simulink model "kinematicstest"  (R2018b)
settings: Solver=ode4  StartTime=0.0  StopTime=40  FixedStep=0.02  RelTol=1e-3
InitFcn:
  | kinematics_initial;
values from neighbouring files (symbols this model uses):
  b = 10.097    [kinematics_initial.m]
  cbar = 1.493520000000000    (= 1.49352)    [kinematics_initial.m]
  J = [948.0 0 0 ... (first row only)    [kinematics_initial.m]
  J_inv = inv(J)    [kinematics_initial.m]
  m = 1454.0*0.453592    (= 659.522768)    [kinematics_initial.m]
  omega_0 = [0;0;0]    [kinematics_initial.m]
  quaternion0 = angle2quat(euler0(3), euler0(2), euler0(1))    [kinematics_initial.m]
  VI0 = [40;0;0]    [kinematics_initial.m]
  XI0 = [0;0;-7]    [kinematics_initial.m]
undefined symbols (not defined in the file or in its folder): C172, current_CG_position, magnitude, QTG_C172
libraries: aerolibasang x3, aerolibtransform2 x2, aerolibatmos2 x2, sharedtransform x2, aerolibconvert2 x1, dspmtrx3 x1, sharedutil x1
settings Model: Creator=arthus  LastModifiedBy=arthus

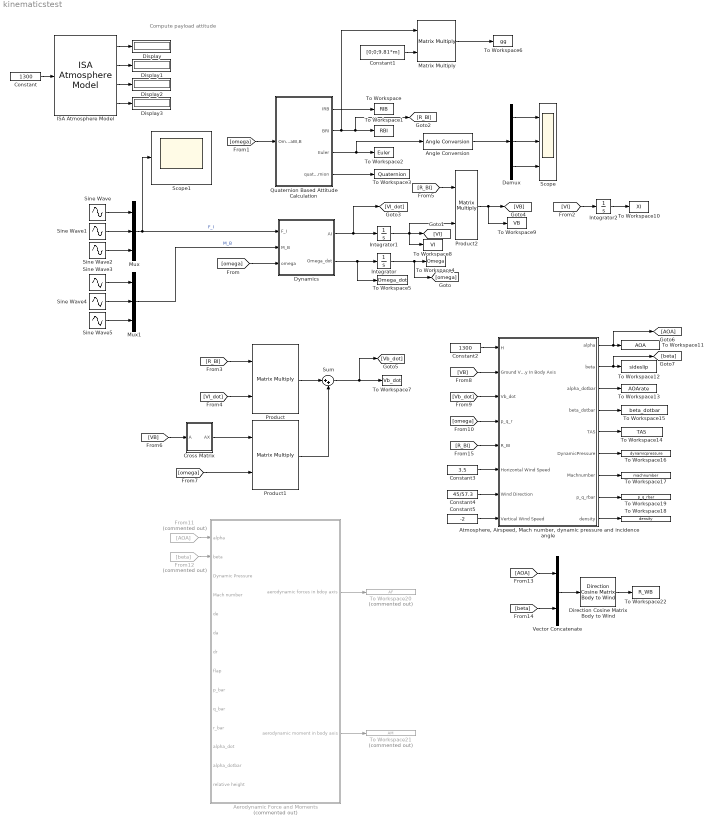
== system kinematicstest ==
  note: Compute payload attitude
  Aerodynamic Force and Moments : Subsystem  Commented=on
  Angle Conversion : aerolibconvert2/Angle Conversion  IU=rad  OU=deg
  "Atmosphere, Airspeed, Mach number, dynamic pressure and incidence angle " : Subsystem
  Constant : Constant  Value=1300
  Constant1 : Constant  Value=[0;0;9.81*m]  VectorParams1D=off
  Constant2 : Constant  Value=1300
  Constant3 : Constant  Value=3.5
  Constant4 : Constant  Value=45/57.3
  Constant5 : Constant  Value=-2
  Cross Matrix : Subsystem
  Demux : Demux  Outputs=3
  Direction Cosine Matrix Body to Wind : aerolibtransform2/Direction Cosine Matrix Body to Wind
      settings: SourceProductName=Aerospace Blockset  SourceProductBaseCode=AE
  Display{,1..3} (4 alike) : Display
  Dynamics : Subsystem
  From11 : From  Commented=on  GotoTag=AOA
  From12 : From  Commented=on  GotoTag=beta
  ISA Atmosphere Model : aerolibatmos2/ISA Atmosphere Model  custom=off  g=9.80665  gamma=1.4  R=287.0531  L=0.0065  h_trop=11000  h_strat=20000  rho0=1.225  P0=101325  T0=288.15  h0=0
      settings: SourceProductName=Aerospace Blockset
  Integrator : Integrator  InitialCondition=omega_0
  Integrator1 : Integrator  InitialCondition=VI0
  Integrator2 : Integrator  InitialCondition=XI0
  Matrix Multiply : Product  Multiplication=Matrix(*)
  Mux : Mux  Inputs=3
  Mux1 : Mux  Inputs=3
  Product : Product  Multiplication=Matrix(*)
  Product1 : Product  Multiplication=Matrix(*)
  Product2 : Product  Multiplication=Matrix(*)
  Quaternion Based Attitude Calculation : Subsystem
  Scope : Scope  NumInputPorts=3
  Scope1 : Scope
  Sine Wave : Sin  Amplitude=0.3  Frequency=pi  SampleTime=0
  Sine Wave1 : Sin  Amplitude=0.1  Frequency=pi  SampleTime=0
  Sine Wave2 : Sin  Amplitude=0.4  Frequency=pi  SampleTime=0
  Sine Wave3 : Sin  Amplitude=0.3  Frequency=pi  SampleTime=0
  Sine Wave4 : Sin  Amplitude=0.1  Frequency=pi  SampleTime=0
  Sine Wave5 : Sin  Amplitude=0.4  Frequency=pi  SampleTime=0
  Sum : Sum  Inputs=|++
  To Workspace : ToWorkspace  VariableName=RIB  SampleTime=-1
  To Workspace1 : ToWorkspace  VariableName=RBI  SampleTime=-1
  To Workspace10 : ToWorkspace  VariableName=XI  SampleTime=-1
  To Workspace11 : ToWorkspace  VariableName=AOA  SampleTime=-1
  To Workspace12 : ToWorkspace  VariableName=sideslip  SampleTime=-1
  To Workspace13 : ToWorkspace  VariableName=AOArate  SampleTime=-1
  To Workspace14 : ToWorkspace  VariableName=TAS  SampleTime=-1
  To Workspace15 : ToWorkspace  VariableName=beta_dotbar  SampleTime=-1
  To Workspace16 : ToWorkspace  VariableName=dynamicpressure  SampleTime=-1
  To Workspace17 : ToWorkspace  VariableName=machnumber  SampleTime=-1
  To Workspace18 : ToWorkspace  VariableName=density  SampleTime=-1
  To Workspace19 : ToWorkspace  VariableName=p_q_rbar  SampleTime=-1
  To Workspace2 : ToWorkspace  VariableName=Euler  SampleTime=-1
  To Workspace20 : ToWorkspace  Commented=on  VariableName=AF  SampleTime=-1
  To Workspace21 : ToWorkspace  Commented=on  VariableName=AM  SampleTime=-1
  To Workspace22 : ToWorkspace  VariableName=R_WB  SampleTime=-1
  To Workspace3 : ToWorkspace  VariableName=Quaternion  SampleTime=-1
  To Workspace4 : ToWorkspace  VariableName=Omega  SampleTime=-1
  To Workspace5 : ToWorkspace  VariableName=Omega_dot  SampleTime=-1
  To Workspace6 : ToWorkspace  VariableName=gg  SampleTime=-1
  To Workspace7 : ToWorkspace  VariableName=Vb_dot  SampleTime=-1
  To Workspace8 : ToWorkspace  VariableName=VI  SampleTime=-1
  To Workspace9 : ToWorkspace  VariableName=VB  SampleTime=-1
  Vector Concatenate : Concatenate
  wires:
  Quaternion Based Attitude Calculation/3(Euler) -> Angle Conversion/1, To Workspace2/1
  Quaternion Based Attitude Calculation/2(BRI) -> Matrix Multiply/1, [R_BI], To Workspace1/1
  Quaternion Based Attitude Calculation/1(IRB) -> To Workspace/1
  Quaternion Based Attitude Calculation/4(quaternion) -> To Workspace3/1
  Sine Wave/1 -> Mux/1
  Sine Wave1/1 -> Mux/2
  Sine Wave2/1 -> Mux/3
  Demux/1 -> Scope/1
  Demux/2 -> Scope/2
  Demux/3 -> Scope/3
  Angle Conversion/1 -> Demux/1
  Constant/1 -> ISA Atmosphere Model/1
  ISA Atmosphere Model/1 -> Display/1
  ISA Atmosphere Model/2 -> Display1/1
  ISA Atmosphere Model/3 -> Display2/1
  ISA Atmosphere Model/4 -> Display3/1
  Constant1/1 -> Matrix Multiply/2
  Matrix Multiply/1 -> To Workspace6/1
  Dynamics/1(AI) -> [VI_dot], Integrator1/1
  Dynamics/2(Omega_dot) -> To Workspace5/1, Integrator/1
  Integrator1/1 -> To Workspace8/1, Product2/2, [VI]
  Integrator/1 -> [omega], To Workspace4/1
  Mux/1 -> Scope1/1, Dynamics/1(F_I)  "F_I"
  [omega] -> Dynamics/3(omega)
  Sine Wave5/1 -> Mux1/3
  Sine Wave3/1 -> Mux1/1
  Sine Wave4/1 -> Mux1/2
  Mux1/1 -> Dynamics/2(M_B)  "M_B"
  [omega] -> Quaternion Based Attitude Calculation/1(OmegaBI,B)
  [VI_dot] -> Product/2
  [R_BI] -> Product/1
  Product/1 -> Sum/1
  Sum/1 -> [Vb_dot], To Workspace7/1
  Cross Matrix/1(AX) -> Product1/1
  [R_BI] -> Product2/1
  Product2/1 -> To Workspace9/1, [VB]
  [VB] -> Cross Matrix/1(A)
  [omega] -> Product1/2
  Product1/1 -> Sum/2
  [VI] -> Integrator2/1
  Integrator2/1 -> To Workspace10/1
  Constant2/1 -> "Atmosphere, Airspeed, Mach number, dynamic pressure and incidence angle "/1(H)
  [VB] -> "Atmosphere, Airspeed, Mach number, dynamic pressure and incidence angle "/2(Ground Velocity In Body Axis)
  [Vb_dot] -> "Atmosphere, Airspeed, Mach number, dynamic pressure and incidence angle "/3(Vb_dot)
  [omega] -> "Atmosphere, Airspeed, Mach number, dynamic pressure and incidence angle "/4(p_q_r)
  "Atmosphere, Airspeed, Mach number, dynamic pressure and incidence angle "/1(alpha) -> [AOA], To Workspace11/1
  "Atmosphere, Airspeed, Mach number, dynamic pressure and incidence angle "/2(beta) -> [beta], To Workspace12/1
  "Atmosphere, Airspeed, Mach number, dynamic pressure and incidence angle "/3(alpha_dotbar) -> To Workspace13/1
  "Atmosphere, Airspeed, Mach number, dynamic pressure and incidence angle "/5(TAS) -> To Workspace14/1
  "Atmosphere, Airspeed, Mach number, dynamic pressure and incidence angle "/4(beta_dotbar) -> To Workspace15/1
  "Atmosphere, Airspeed, Mach number, dynamic pressure and incidence angle "/6(DynamicPressure) -> To Workspace16/1
  "Atmosphere, Airspeed, Mach number, dynamic pressure and incidence angle "/7(Machnumber) -> To Workspace17/1
  "Atmosphere, Airspeed, Mach number, dynamic pressure and incidence angle "/9(density) -> To Workspace18/1
  "Atmosphere, Airspeed, Mach number, dynamic pressure and incidence angle "/8(p_q_rbar) -> To Workspace19/1
  Aerodynamic Force and Moments/1(aerodynamic forces in bdoy axis) -> To Workspace20/1
  Aerodynamic Force and Moments/2(aerodynamic moment in body axis) -> To Workspace21/1
  From11/1 -> Aerodynamic Force and Moments/1(alpha)
  From12/1 -> Aerodynamic Force and Moments/2(beta)
  Vector Concatenate/1 -> Direction Cosine Matrix Body to Wind/1
  [AOA] -> Vector Concatenate/1
  [beta] -> Vector Concatenate/2
  Direction Cosine Matrix Body to Wind/1 -> To Workspace22/1
  [R_BI] -> "Atmosphere, Airspeed, Mach number, dynamic pressure and incidence angle "/5(R_BI)
  Constant3/1 -> "Atmosphere, Airspeed, Mach number, dynamic pressure and incidence angle "/6(Horizontal Wind Speed)
  Constant4/1 -> "Atmosphere, Airspeed, Mach number, dynamic pressure and incidence angle "/7(Wind Direction)
  Constant5/1 -> "Atmosphere, Airspeed, Mach number, dynamic pressure and incidence angle "/8(Vertical Wind Speed)

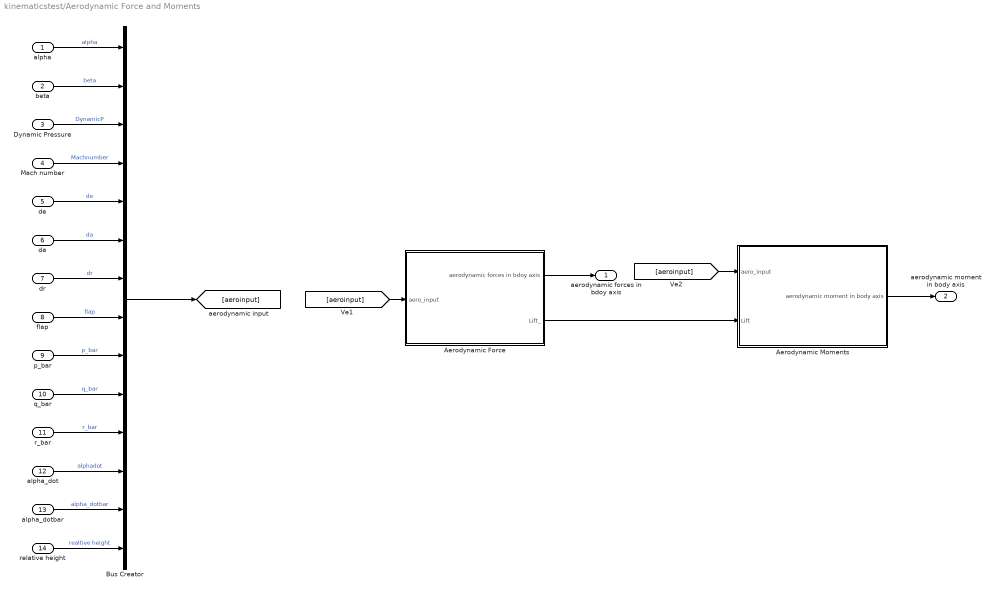
== system kinematicstest/Aerodynamic Force and Moments ==
  alpha : Inport
  beta : Inport  Port=2
  Dynamic Pressure : Inport  Port=3
  Mach number : Inport  Port=4
  de : Inport  Port=5
  da : Inport  Port=6
  dr : Inport  Port=7
  flap : Inport  Port=8
  p_bar : Inport  Port=9
  q_bar : Inport  Port=10
  r_bar : Inport  Port=11
  alpha_dot : Inport  Port=12
  alpha_dotbar : Inport  Port=13
  relative height : Inport  Port=14
  "Aerodynamic Force " : Subsystem  mask(Calculate Aerodynamic Forces in body axis){referenceaera=C172.Geometry.wingarea}
      mask prompts: referenceaera "Wing Aera"
  Aerodynamic Moments : Subsystem  mask(Calculate Aerodynamic Moments in body axis){referenceaera=C172.Geometry.wingarea, meanchord=C172.Geometry.chord, span=C172.Geometry.wingspan}
  Bus Creator : BusCreator  Inputs=14
  aerodynamic forces in bdoy axis : Outport
  aerodynamic moment in body axis : Outport  Port=2
  wires:
  alpha/1 -> Bus Creator/1  "alpha"
  beta/1 -> Bus Creator/2  "beta"
  Dynamic Pressure/1 -> Bus Creator/3  "DynamicP"
  Mach number/1 -> Bus Creator/4  "Machnumber"
  de/1 -> Bus Creator/5  "de"
  da/1 -> Bus Creator/6  "da"
  dr/1 -> Bus Creator/7  "dr"
  flap/1 -> Bus Creator/8  "flap"
  Bus Creator/1 -> [aeroinput]
  p_bar/1 -> Bus Creator/9  "p_bar"
  q_bar/1 -> Bus Creator/10  "q_bar"
  r_bar/1 -> Bus Creator/11  "r_bar"
  alpha_dot/1 -> Bus Creator/12  "alphadot"
  alpha_dotbar/1 -> Bus Creator/13  "alpha_dotbar"
  "Aerodynamic Force "/1(aerodynamic forces in bdoy axis) -> aerodynamic forces in bdoy axis/1
  Aerodynamic Moments/1(aerodynamic moment in body axis) -> aerodynamic moment in body axis/1
  [aeroinput] -> "Aerodynamic Force "/1(aero_input)
  [aeroinput] -> Aerodynamic Moments/1(aero_input)
  relative height/1 -> Bus Creator/14  "realtive height"
  "Aerodynamic Force "/2(Lift_) -> Aerodynamic Moments/2(Lift)

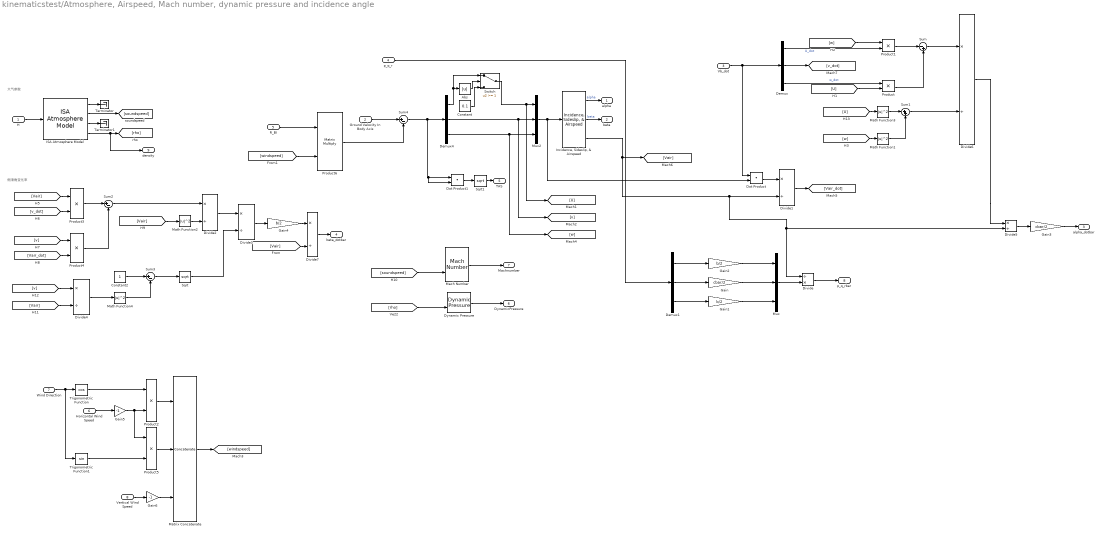
== system kinematicstest/Atmosphere, Airspeed, Mach number, dynamic pressure and incidence angle  ==
  note: 侧滑角变化率
  note: 大气参数
  H : Inport
  Ground Velocity In Body Axis : Inport  Port=2
  Vb_dot : Inport  Port=3
  p_q_r : Inport  Port=4
  R_BI : Inport  Port=5
  Horizontal Wind Speed : Inport  Port=6
  Wind Direction : Inport  Port=7
  Vertical Wind Speed : Inport  Port=8
  Abs : Abs
  Constant : Constant  Value=0.1
  Constant2 : Constant
  Demux : Demux  Outputs=3
  Demux1 : Demux  Outputs=3
  Demux4 : Demux  Outputs=3
  Divide : Product  Inputs=/*
  Divide{1..7} (7 alike) : Product  Inputs=*/
  Dot Product : DotProduct  InputSameDT=on  OutDataTypeStr=Inherit: Inherit via internal rule
  Dot Product1 : DotProduct  InputSameDT=on  OutDataTypeStr=Inherit: Inherit via internal rule
  Dynamic Pressure : aerolibasang/Dynamic Pressure
  Gain : Gain  Gain=cbar/2
  Gain1 : Gain  Gain=b/2
  Gain2 : Gain  Gain=b/2
  Gain3 : Gain  Gain=cbar/2
  Gain4 : Gain  Gain=b/2
  Gain5 : Gain  Gain=-1
  Gain6 : Gain  Gain=-1
  ISA Atmosphere Model : aerolibatmos2/ISA Atmosphere Model  custom=off  g=9.80665  gamma=1.4  R=287.0531  L=0.0065  h_trop=11000  h_strat=20000  rho0=1.225  P0=101325  T0=288.15  h0=0
      settings: SourceProductName=Aerospace Blockset
  "Incidence, Sideslip, & Airspeed" : aerolibasang/Incidence, Sideslip, & Airspeed
      settings: SourceProductName=Aerospace Blockset
  Mach Number : aerolibasang/Mach Number
      settings: SourceProductName=Aerospace Blockset  SourceProductBaseCode=AE
  Math Function{1..4} (4 alike) : Math  Operator=magnitude^2  SaturateOnIntegerOverflow=on
  Matrix Concatenate : Concatenate  NumInputs=3  Mode=Multidimensional array
  Mux : Mux  Inputs=3
  Mux2 : Mux  Inputs=3
  Product{,1,3..4} (4 alike) : Product  RndMeth=Zero
  Product2 : Product
  Product5 : Product
  Product6 : Product  Multiplication=Matrix(*)
  Sqrt : Sqrt  SaturateOnIntegerOverflow=on
  Sqrt1 : Sqrt  SaturateOnIntegerOverflow=on
  Sum : Sum  Inputs=|-+
  Sum1 : Sum  Inputs=|++
  Sum2 : Sum  Inputs=|+-
  Sum3 : Sum  Inputs=|+-
  Sum4 : Sum  Inputs=|+-
  Switch : Switch  Threshold=1
  Terminator : Terminator
  Terminator1 : Terminator
  Trigonometric Function : Trigonometry  Operator=cos
  Trigonometric Function1 : Trigonometry
  alpha : Outport
  beta : Outport  Port=2
  alpha_dotbar : Outport  Port=3
  beta_dotbar : Outport  Port=4
  TAS : Outport  Port=5
  DynamicPressure : Outport  Port=6
  Machnumber : Outport  Port=7
  p_q_rbar : Outport  Port=8
  density : Outport  Port=9
  wires:
  "Incidence, Sideslip, & Airspeed"/2 -> beta/1  "beta"
  "Incidence, Sideslip, & Airspeed"/1 -> alpha/1  "alpha"
  "Incidence, Sideslip, & Airspeed"/3 -> Divide1/2, Divide/1, Divide5/2, [Vair]
  Mux2/1 -> "Incidence, Sideslip, & Airspeed"/1, Dot Product/2
  Demux4/2 -> Mux2/2, [v]
  Demux4/3 -> Mux2/3, [w]
  Abs/1 -> Switch/2
  Switch/1 -> Mux2/1, [U]
  Demux4/1 -> Abs/1, Switch/1
  Constant/1 -> Switch/3
  ISA Atmosphere Model/1 -> Terminator/1
  ISA Atmosphere Model/3 -> Terminator1/1
  ISA Atmosphere Model/2 -> [soundspeed]
  ISA Atmosphere Model/4 -> density/1, [rho]
  H/1 -> ISA Atmosphere Model/1
  [soundspeed] -> Mach Number/2
  Mach Number/1 -> Machnumber/1
  Dynamic Pressure/1 -> DynamicPressure/1
  [rho] -> Dynamic Pressure/2
  Demux/1 -> Product1/2  "U_dot"
  Demux/2 -> [v_dot]
  Demux/3 -> Product/1  "w_dot"
  [U] -> Product/2
  Product/1 -> Sum/2
  [w] -> Product1/1
  Product1/1 -> Sum/1
  Sum/1 -> Divide6/1
  Math Function3/1 -> Sum1/1
  [Vair] -> Product3/1
  [v_dot] -> Product3/2
  Product3/1 -> Sum2/1
  [v] -> Product4/1
  [Vair_dot] -> Product4/2
  Product4/1 -> Sum2/2
  Dot Product/1 -> Divide1/1
  Divide1/1 -> [Vair_dot]
  Sum2/1 -> Divide2/1
  Math Function2/1 -> Divide2/2
  [Vair] -> Math Function2/1
  Divide2/1 -> Divide3/1
  Sqrt/1 -> Divide3/2
  Sum3/1 -> Sqrt/1
  Constant2/1 -> Sum3/1
  Math Function4/1 -> Sum3/2
  Divide4/1 -> Math Function4/1
  [Vair] -> Divide4/2
  [v] -> Divide4/1
  Divide3/1 -> Gain4/1
  [U] -> Math Function3/1
  Sum1/1 -> Divide6/2
  [w] -> Math Function1/1
  Math Function1/1 -> Sum1/2
  Vb_dot/1 -> Demux/1, Dot Product/1
  Dot Product1/1 -> Sqrt1/1
  Sqrt1/1 -> TAS/1
  Demux1/2 -> Gain/1
  Demux1/3 -> Gain1/1
  Demux1/1 -> Gain2/1
  Gain2/1 -> Mux/1
  Gain/1 -> Mux/2
  Gain1/1 -> Mux/3
  Mux/1 -> Divide/2
  Divide/1 -> p_q_rbar/1
  Divide5/1 -> Gain3/1
  Gain3/1 -> alpha_dotbar/1
  p_q_r/1 -> Demux1/1
  Divide6/1 -> Divide5/1
  Gain4/1 -> Divide7/1
  Divide7/1 -> beta_dotbar/1
  [Vair] -> Divide7/2
  R_BI/1 -> Product6/1
  Wind Direction/1 -> Trigonometric Function1/1, Trigonometric Function/1
  Trigonometric Function/1 -> Product2/1
  Horizontal Wind Speed/1 -> Gain5/1
  Trigonometric Function1/1 -> Product5/2
  Gain5/1 -> Product5/1, Product2/2
  Vertical Wind Speed/1 -> Gain6/1
  Product2/1 -> Matrix Concatenate/1
  Product5/1 -> Matrix Concatenate/2
  Gain6/1 -> Matrix Concatenate/3
  Matrix Concatenate/1 -> [windspeed]
  [windspeed] -> Product6/2
  Sum4/1 -> Dot Product1/2, Dot Product1/1, Demux4/1
  Product6/1 -> Sum4/2
  Ground Velocity In Body Axis/1 -> Sum4/1

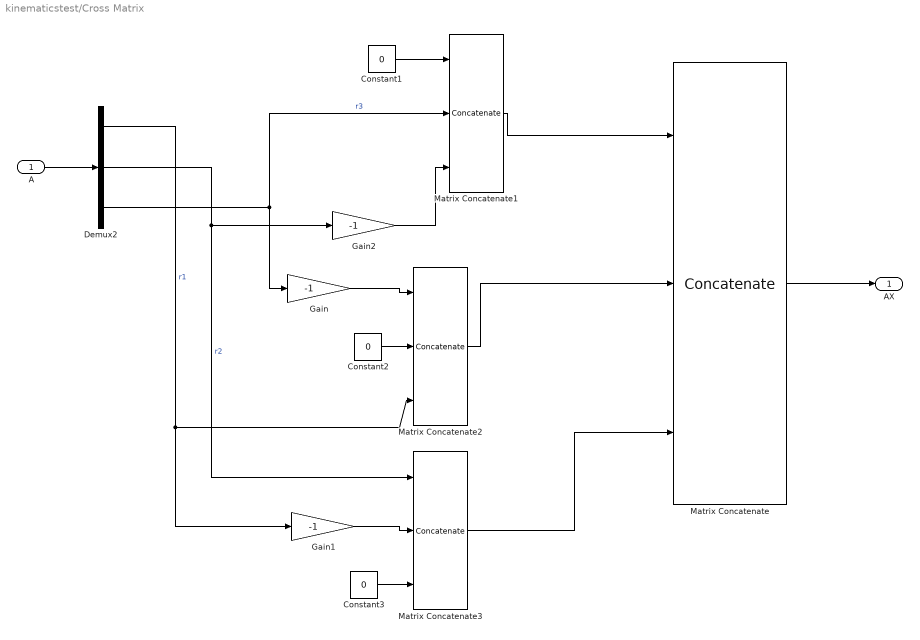
== system kinematicstest/Cross Matrix ==
  A : Inport
  Constant1 : Constant  Value=0  VectorParams1D=off
  Constant2 : Constant  Value=0  VectorParams1D=off
  Constant3 : Constant  Value=0  VectorParams1D=off
  Demux2 : Demux  Outputs=3
  Gain : Gain  Gain=-1
  Gain1 : Gain  Gain=-1
  Gain2 : Gain  Gain=-1
  Matrix Concatenate : Concatenate  NumInputs=3  Mode=Multidimensional array  ConcatenateDimension=2
  Matrix Concatenate1 : Concatenate  NumInputs=3  Mode=Multidimensional array
  Matrix Concatenate2 : Concatenate  NumInputs=3  Mode=Multidimensional array
  Matrix Concatenate3 : Concatenate  NumInputs=3  Mode=Multidimensional array
  AX : Outport
  wires:
  A/1 -> Demux2/1
  Demux2/1 -> Gain1/1, Matrix Concatenate2/3  "r1"
  Demux2/2 -> Gain2/1, Matrix Concatenate3/1  "r2"
  Matrix Concatenate/1 -> AX/1
  Demux2/3 -> Gain/1, Matrix Concatenate1/2  "r3"
  Matrix Concatenate1/1 -> Matrix Concatenate/1
  Matrix Concatenate2/1 -> Matrix Concatenate/2
  Constant2/1 -> Matrix Concatenate2/2
  Gain/1 -> Matrix Concatenate2/1
  Matrix Concatenate3/1 -> Matrix Concatenate/3
  Gain1/1 -> Matrix Concatenate3/2
  Constant3/1 -> Matrix Concatenate3/3
  Constant1/1 -> Matrix Concatenate1/1
  Gain2/1 -> Matrix Concatenate1/3

== system kinematicstest/Dynamics ==
  F_I : Inport
  M_B : Inport  Port=2
  omega : Inport  Port=3
  Cross Matrix : Subsystem
  Gain : Gain  Gain=1/m
  Gain1 : Gain  Gain=J_inv  Multiplication=Matrix(K*u)
  Gain2 : Gain  Gain=J  Multiplication=Matrix(K*u)
  Product : Product  Multiplication=Matrix(*)
  Sum : Sum  Inputs=|+-
  AI : Outport
  Omega_dot : Outport  Port=2
  wires:
  Gain/1 -> AI/1
  F_I/1 -> Gain/1
  Sum/1 -> Gain1/1
  Gain1/1 -> Omega_dot/1
  M_B/1 -> Sum/1
  omega/1 -> Product/2, Cross Matrix/1(A)
  Cross Matrix/1(AX) -> Gain2/1
  Gain2/1 -> Product/1
  Product/1 -> Sum/2

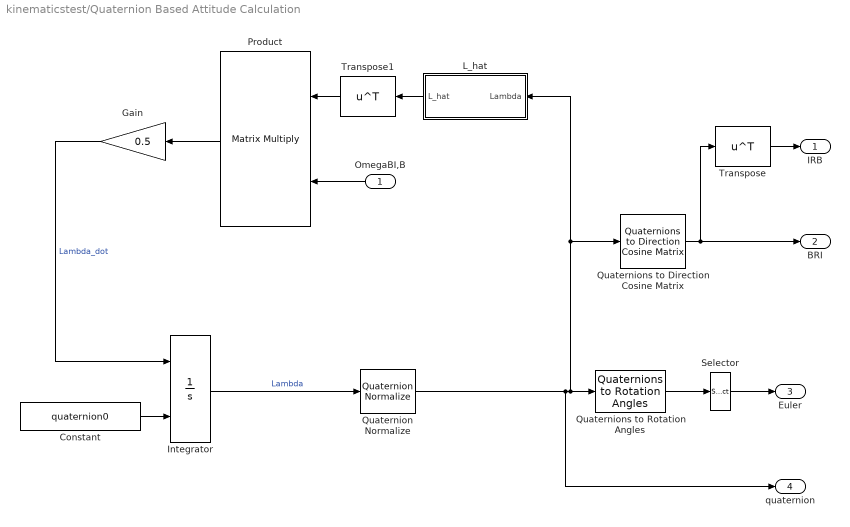
== system kinematicstest/Quaternion Based Attitude Calculation ==
  OmegaBI,B : Inport
  Constant : Constant  Value=quaternion0
  Gain : Gain  Gain=0.5
  Integrator : Integrator  InitialConditionSource=external
  L_hat : Subsystem
  Product : Product  Multiplication=Matrix(*)  RndMeth=Zero
  Quaternion Normalize : sharedutil/Quaternion Normalize  aMode=aMode
      settings: SourceProductName=Aerospace Blockset  SourceProductBaseCode=AE
  Quaternions to Direction Cosine Matrix : sharedtransform/Quaternions to  Direction Cosine Matrix  aMode=aMode
      settings: SourceProductName=Aerospace Blockset  SourceProductBaseCode=AE
  Quaternions to Rotation Angles : sharedtransform/Quaternions to Rotation Angles  rotationOrder=ZYX  aMode=aMode
      settings: SourceProductBaseCode=AE
  Selector : Selector  InputPortWidth=3  IndexOptions=Index vector (dialog)  Indices=[3 2 1]  OutputSizes=1
  Transpose : Math  Operator=transpose  SaturateOnIntegerOverflow=on
  Transpose1 : Math  Operator=transpose  SaturateOnIntegerOverflow=on
  IRB : Outport
  BRI : Outport  Port=2
  Euler : Outport  Port=3
  quaternion : Outport  Port=4
  wires:
  Constant/1 -> Integrator/2
  Quaternions to Rotation Angles/1 -> Selector/1
  Selector/1 -> Euler/1
  Integrator/1 -> Quaternion Normalize/1  "Lambda"
  Gain/1 -> Integrator/1  "Lambda_dot"
  Quaternions to Direction Cosine Matrix/1 -> BRI/1, Transpose/1
  Transpose/1 -> IRB/1
  L_hat/1(L_hat) -> Transpose1/1
  Transpose1/1 -> Product/1
  OmegaBI,B/1 -> Product/2
  Product/1 -> Gain/1
  Quaternion Normalize/1 -> Quaternions to Rotation Angles/1, Quaternions to Direction Cosine Matrix/1, L_hat/1(Lambda), quaternion/1

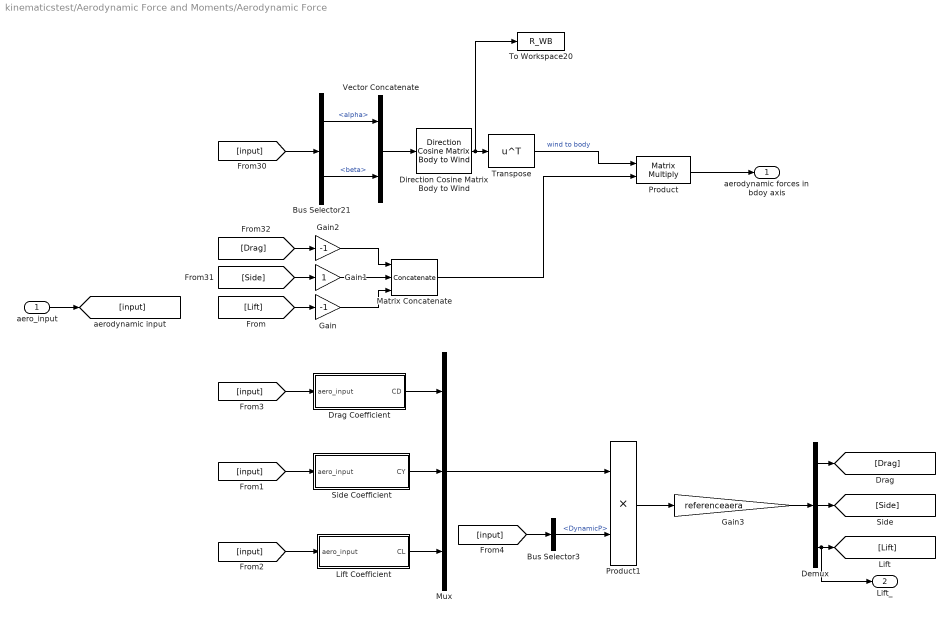
== system kinematicstest/Aerodynamic Force and Moments/Aerodynamic Force  ==
  aero_input : Inport
  Bus Selector21 : BusSelector  OutputSignals=alpha,beta
  Bus Selector3 : BusSelector  OutputSignals=DynamicP
  Demux : Demux  Outputs=3
  Direction Cosine Matrix Body to Wind : aerolibtransform2/Direction Cosine Matrix Body to Wind
      settings: SourceProductName=Aerospace Blockset  SourceProductBaseCode=AE
  Drag Coefficient : Subsystem
  Gain : Gain  Gain=-1
  Gain1 : Gain
  Gain2 : Gain  Gain=-1
  Gain3 : Gain  Gain=referenceaera
  Lift Coefficient : Subsystem
  Matrix Concatenate : Concatenate  NumInputs=3  Mode=Multidimensional array
  Mux : Mux  Inputs=3
  Product : Product  Multiplication=Matrix(*)  RndMeth=Zero
  Product1 : Product  RndMeth=Zero
  Side Coefficient : Subsystem
  To Workspace20 : ToWorkspace  VariableName=R_WB  SampleTime=-1
  Transpose : Math  Operator=transpose  SaturateOnIntegerOverflow=on
  Vector Concatenate : Concatenate
  aerodynamic forces in bdoy axis : Outport
  Lift_ : Outport  Port=2
  wires:
  Transpose/1 -> Product/1  "wind to body"
  Direction Cosine Matrix Body to Wind/1 -> To Workspace20/1, Transpose/1
  Matrix Concatenate/1 -> Product/2
  Gain2/1 -> Matrix Concatenate/1
  [Drag] -> Gain2/1
  Gain1/1 -> Matrix Concatenate/2
  [Side] -> Gain1/1
  Gain/1 -> Matrix Concatenate/3
  [Lift] -> Gain/1
  Vector Concatenate/1 -> Direction Cosine Matrix Body to Wind/1
  Bus Selector21/1 -> Vector Concatenate/1  "<alpha>"
  Bus Selector21/2 -> Vector Concatenate/2  "<beta>"
  [input] -> Bus Selector21/1
  aero_input/1 -> [input]
  [input] -> Bus Selector3/1
  Bus Selector3/1 -> Product1/2  "<DynamicP>"
  Product1/1 -> Gain3/1
  Mux/1 -> Product1/1
  Gain3/1 -> Demux/1
  Demux/1 -> [Drag]
  Demux/2 -> [Side]
  Demux/3 -> Lift_/1, [Lift]
  Product/1 -> aerodynamic forces in bdoy axis/1
  Drag Coefficient/1(CD) -> Mux/1
  Side Coefficient/1(CY) -> Mux/2
  [input] -> Lift Coefficient/1(aero_input)
  [input] -> Side Coefficient/1(aero_input)
  Lift Coefficient/1(CL) -> Mux/3
  [input] -> Drag Coefficient/1(aero_input)

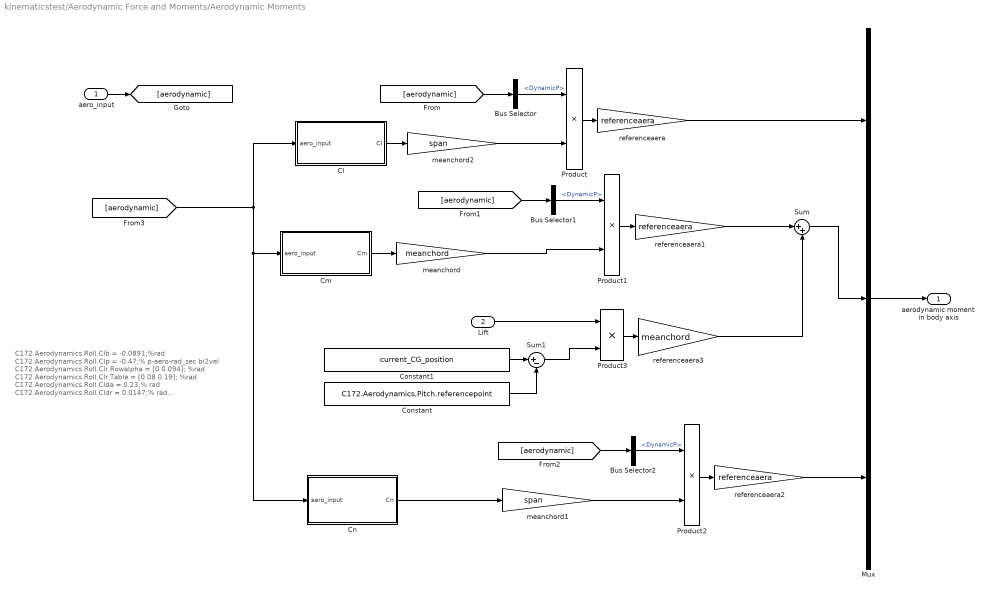
== system kinematicstest/Aerodynamic Force and Moments/Aerodynamic Moments ==
  note: C172.Aerodynamics.Roll.Clb = -0.0891;%rad
      | C172.Aerodynamics.Roll.Clp = -0.47;% p-aero-rad_sec bi2vel
      | C172.Aerodynamics.Roll.Clr.Rowalpha = [0 0.094];  %rad
      | C172.Aerodynamics.Roll.Clr.Table = [0.08 0.19];   %rad
      | C172.Aerodynamics.Roll.Clda = 0.23;% rad
      | C172.Aerodynamics.Roll.Cldr = 0.0147;% rad
      | C172.Aerodynamics.Pitch.Cmalpha = -1.8;% alpha-rad
      | C172.Aerodynamics.Pitch.CmDf.RowFlap = [0 10 20 30];%deg
      | C172.Aerodynamics.Pitch.CmDf.Table = [0 -0.03 -0.05 -0.06];%
      | C172.Aerodynamics.Pitch.CmDf.Type = 'Delta Pitch Moment';
      | C172.Aerodynamics.Pitch.Cmq = -12.4; % q-aero-rad_sec ci2vel
      | C172.Aerodynamics.Pitch.Cmadot = -5.2; % alphadot-rad_sec
      | C172.Aerodynamics.Pitch.Cm0 = 0.1; %
      | C172.Aerodynamics.Pitch.Cmde = -1.28; % elevator-pos-rad
      | C172.Aerodynamics.Yaw.Cnb = 0.0650;% rad
      | C172.Aerodynamics.Yaw.Cnp = -0.03;% p-aero-rad_sec bi2vel
      | C172.Aerodynamics.Yaw.Cnr = -0.099;%  r-aero-rad_sec bi2vel
      | C172.Aerodynamics.Yaw.Cnda = 0.0053;% rad
      | C172.Aerodynamics.Yaw.Cndr = -0.043;% rad
  aero_input : Inport
  Lift : Inport  Port=2
  Bus Selector : BusSelector  OutputSignals=DynamicP
  Bus Selector1 : BusSelector  OutputSignals=DynamicP
  Bus Selector2 : BusSelector  OutputSignals=DynamicP
  Cl : Subsystem
  Cm : Subsystem
  Cn : Subsystem
  Constant : Constant  Value=C172.Aerodynamics.Pitch.referencepoint
  Constant1 : Constant  Value=current_CG_position
  Mux : Mux  Inputs=3
  Product : Product  RndMeth=Zero
  Product1 : Product  RndMeth=Zero
  Product2 : Product  RndMeth=Zero
  Product3 : Product
  Sum : Sum  Inputs=|++
  Sum1 : Sum  Inputs=|+-
  meanchord : Gain  Gain=meanchord
  meanchord1 : Gain  Gain=span
  meanchord2 : Gain  Gain=span
  referenceaera : Gain  Gain=referenceaera
  referenceaera1 : Gain  Gain=referenceaera
  referenceaera2 : Gain  Gain=referenceaera
  referenceaera3 : Gain  Gain=meanchord
  aerodynamic moment in body axis : Outport
  wires:
  Product/1 -> referenceaera/1
  Bus Selector/1 -> Product/1  "<DynamicP>"
  Cn/1(Cn) -> meanchord1/1
  aero_input/1 -> [aerodynamic]
  Cm/1(Cm) -> meanchord/1
  [aerodynamic] -> Cn/1(aero_input), Cm/1(aero_input), Cl/1(aero_input)
  Cl/1(Cl) -> meanchord2/1
  [aerodynamic] -> Bus Selector/1
  Mux/1 -> aerodynamic moment in body axis/1
  meanchord2/1 -> Product/2
  referenceaera/1 -> Mux/1
  Product1/1 -> referenceaera1/1
  Bus Selector1/1 -> Product1/1  "<DynamicP>"
  [aerodynamic] -> Bus Selector1/1
  meanchord/1 -> Product1/2
  Product2/1 -> referenceaera2/1
  Bus Selector2/1 -> Product2/1  "<DynamicP>"
  [aerodynamic] -> Bus Selector2/1
  referenceaera1/1 -> Sum/1
  Sum/1 -> Mux/2
  referenceaera3/1 -> Sum/2
  referenceaera2/1 -> Mux/3
  meanchord1/1 -> Product2/2
  Constant1/1 -> Sum1/1
  Constant/1 -> Sum1/2
  Product3/1 -> referenceaera3/1
  Lift/1 -> Product3/1
  Sum1/1 -> Product3/2

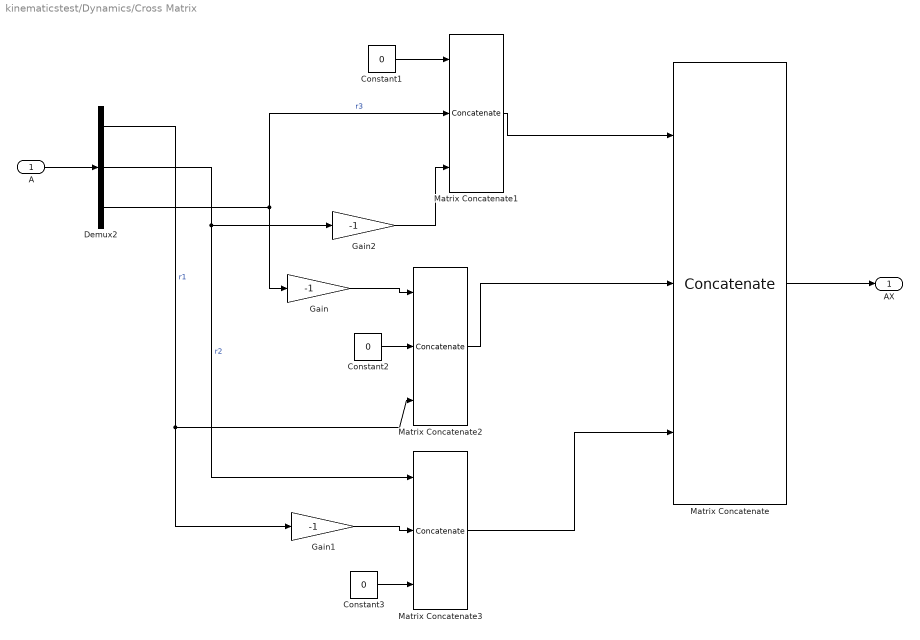
== system kinematicstest/Dynamics/Cross Matrix ==
  A : Inport
  Constant1 : Constant  Value=0  VectorParams1D=off
  Constant2 : Constant  Value=0  VectorParams1D=off
  Constant3 : Constant  Value=0  VectorParams1D=off
  Demux2 : Demux  Outputs=3
  Gain : Gain  Gain=-1
  Gain1 : Gain  Gain=-1
  Gain2 : Gain  Gain=-1
  Matrix Concatenate : Concatenate  NumInputs=3  Mode=Multidimensional array  ConcatenateDimension=2
  Matrix Concatenate1 : Concatenate  NumInputs=3  Mode=Multidimensional array
  Matrix Concatenate2 : Concatenate  NumInputs=3  Mode=Multidimensional array
  Matrix Concatenate3 : Concatenate  NumInputs=3  Mode=Multidimensional array
  AX : Outport
  wires:
  A/1 -> Demux2/1
  Demux2/1 -> Gain1/1, Matrix Concatenate2/3  "r1"
  Demux2/2 -> Gain2/1, Matrix Concatenate3/1  "r2"
  Matrix Concatenate/1 -> AX/1
  Demux2/3 -> Gain/1, Matrix Concatenate1/2  "r3"
  Matrix Concatenate1/1 -> Matrix Concatenate/1
  Matrix Concatenate2/1 -> Matrix Concatenate/2
  Constant2/1 -> Matrix Concatenate2/2
  Gain/1 -> Matrix Concatenate2/1
  Matrix Concatenate3/1 -> Matrix Concatenate/3
  Gain1/1 -> Matrix Concatenate3/2
  Constant3/1 -> Matrix Concatenate3/3
  Constant1/1 -> Matrix Concatenate1/1
  Gain2/1 -> Matrix Concatenate1/3

== system kinematicstest/Quaternion Based Attitude Calculation/L_hat ==
  Lambda : Inport
  Create Diagonal Matrix : dspmtrx3/Create Diagonal Matrix
      settings: SourceProductName=DSP System Toolbox  SourceProductBaseCode=DS
  Cross Matrix : Subsystem
  Gain : Gain  Gain=-1
  Gain1 : Gain  Gain=[1 1 1]
  Gain2 : Gain  Gain=-1
  Matrix Concatenate : Concatenate  Mode=Multidimensional array  ConcatenateDimension=2
  Selector : Selector  InputPortWidth=4  IndexOptions=Index vector (dialog)  Indices=[2 3 4]  OutputSizes=1
  Selector1 : Selector  InputPortWidth=4  IndexOptions=Index vector (dialog)  Indices=[1]  OutputSizes=1
  Sum : Sum  Inputs=|++
  L_hat : Outport
  wires:
  Lambda/1 -> Selector/1, Selector1/1
  Gain/1 -> Matrix Concatenate/1
  Matrix Concatenate/1 -> L_hat/1
  Cross Matrix/1(AX) -> Gain2/1  "LambdaX"
  Sum/1 -> Matrix Concatenate/2
  Selector1/1 -> Gain1/1
  Gain1/1 -> Create Diagonal Matrix/1
  Selector/1 -> Cross Matrix/1(A), Gain/1
  Create Diagonal Matrix/1 -> Sum/2
  Gain2/1 -> Sum/1

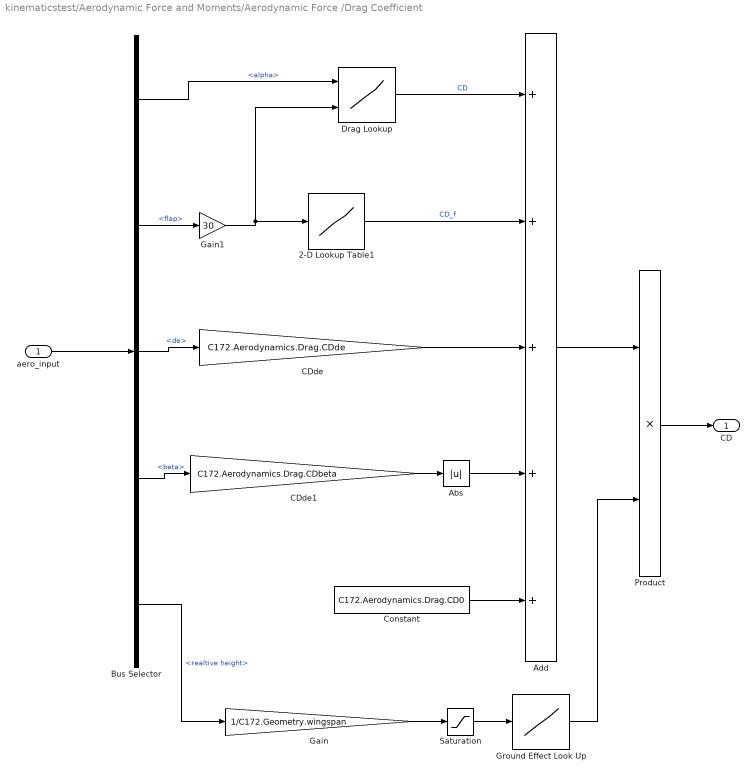
== system kinematicstest/Aerodynamic Force and Moments/Aerodynamic Force /Drag Coefficient ==
  aero_input : Inport
  2-D Lookup Table1 : Lookup_n-D  NumberOfTableDimensions=1  BreakpointsForDimension1=C172.Aerodynamics.Drag.CDDf.RowFlap  BreakpointsForDimension2=C172.Aerodynamics.Drag.CDwbh.ColumnFlap  Table=C172.Aerodynamics.Drag.CDDf.Table  InternalRulePriority=Speed  RndMeth=Simplest  InputSameDT=on
  Abs : Abs
  Add : Sum  Inputs=+++++
  Bus Selector : BusSelector  OutputSignals=alpha,flap,de,beta,realtive height
  CDde : Gain  Gain=C172.Aerodynamics.Drag.CDde
  CDde1 : Gain  Gain=C172.Aerodynamics.Drag.CDbeta
  Constant : Constant  Value=C172.Aerodynamics.Drag.CD0
  Drag Lookup : Lookup_n-D  BreakpointsForDimension1=C172.Aerodynamics.Drag.CDwbh.RowAlpha  BreakpointsForDimension2=C172.Aerodynamics.Drag.CDwbh.ColumnFlap  Table=C172.Aerodynamics.Drag.CDwbh.Table  InternalRulePriority=Speed  RndMeth=Simplest  InputSameDT=on
  Gain : Gain  Gain=1/C172.Geometry.wingspan
  Gain1 : Gain  Gain=30
  Ground Effect Look Up : Lookup_n-D  NumberOfTableDimensions=1  BreakpointsForDimension1=C172.Aerodynamics.GroundDragEffect.RowHeight  BreakpointsForDimension2=C172.Aerodynamics.Drag.CDwbh.ColumnFlap  Table=C172.Aerodynamics.GroundDragEffect.Table  InternalRulePriority=Speed  RndMeth=Simplest  InputSameDT=on
  Product : Product
  Saturation : Saturate  UpperLimit=1.1  LowerLimit=0
  CD : Outport
  wires:
  Drag Lookup/1 -> Add/1  "CD"
  aero_input/1 -> Bus Selector/1
  Constant/1 -> Add/5
  2-D Lookup Table1/1 -> Add/2  "CD_f"
  CDde1/1 -> Abs/1
  CDde/1 -> Add/3
  Bus Selector/3 -> CDde/1  "<de>"
  Bus Selector/4 -> CDde1/1  "<beta>"
  Abs/1 -> Add/4
  Bus Selector/2 -> Gain1/1  "<flap>"
  Bus Selector/1 -> Drag Lookup/1  "<alpha>"
  Add/1 -> Product/1
  Product/1 -> CD/1
  Ground Effect Look Up/1 -> Product/2
  Bus Selector/5 -> Gain/1  "<realtive height>"
  Saturation/1 -> Ground Effect Look Up/1
  Gain/1 -> Saturation/1
  Gain1/1 -> Drag Lookup/2, 2-D Lookup Table1/1

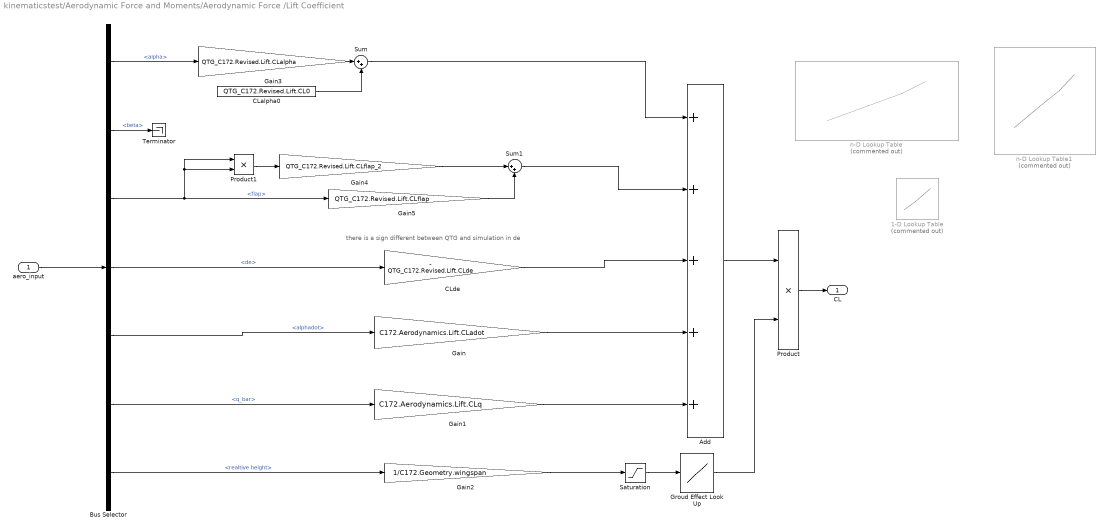
== system kinematicstest/Aerodynamic Force and Moments/Aerodynamic Force /Lift Coefficient ==
  note: there is a sign different between QTG and simulation in de
  aero_input : Inport
  1-D Lookup Table : Lookup_n-D  Commented=on  NumberOfTableDimensions=1  BreakpointsForDimension1=C172.Aerodynamics.Lift.CLDf.RowFlap  Table=C172.Aerodynamics.Lift.CLDf.Table  InternalRulePriority=Speed  RndMeth=Simplest  InputSameDT=on
  Add : Sum  Inputs=+++++
  Bus Selector : BusSelector  OutputSignals=alpha,beta,flap,de,alphadot,q_bar,realtive height
  CLalpha0 : Constant  Value=QTG_C172.Revised.Lift.CL0
  CLde : Gain  Gain=- QTG_C172.Revised.Lift.CLde
  Gain : Gain  Gain=C172.Aerodynamics.Lift.CLadot
  Gain1 : Gain  Gain=C172.Aerodynamics.Lift.CLq
  Gain2 : Gain  Gain=1/C172.Geometry.wingspan
  Gain3 : Gain  Gain=QTG_C172.Revised.Lift.CLalpha
  Gain4 : Gain  Gain=QTG_C172.Revised.Lift.CLflap_2
  Gain5 : Gain  Gain=QTG_C172.Revised.Lift.CLflap
  Groud Effect Look Up : Lookup_n-D  NumberOfTableDimensions=1  BreakpointsForDimension1=C172.Aerodynamics.GroundLiftEffect.RowHeight  Table=C172.Aerodynamics.GroundLiftEffect.Table  InternalRulePriority=Speed  RndMeth=Simplest  InputSameDT=on
  Product : Product
  Product1 : Product
  Saturation : Saturate  UpperLimit=1.1  LowerLimit=0
  Sum : Sum  Inputs=|++
  Sum1 : Sum  Inputs=|++
  Terminator : Terminator
  n-D Lookup Table : Lookup_n-D  Commented=on  BreakpointsForDimension1=C172.Aerodynamics.Lift.CLwbh.RowAlpha  BreakpointsForDimension2=C172.Aerodynamics.Lift.CLwbh.Stall_Hyst_Norm  BreakpointsForDimension3=[5, 7]  Table=C172.Aerodynamics.Lift.CLwbh.Table  InternalRulePriority=Speed  RndMeth=Simplest  InputSameDT=on
  n-D Lookup Table1 : Lookup_n-D  Commented=on  NumberOfTableDimensions=3  BreakpointsForDimension1=C172.Aerodynamics.Lift.CLalpha.RowAlpha  BreakpointsForDimension2=C172.Aerodynamics.Lift.CLalpha.ColumnBeta  BreakpointsForDimension3=C172.Aerodynamics.Lift.CLalpha.PageFlap  Table=C172.Aerodynamics.Lift.CLalpha.Table  InternalRulePriority=Speed  RndMeth=Simplest  InputSameDT=on
  CL : Outport
  wires:
  aero_input/1 -> Bus Selector/1
  Bus Selector/6 -> Gain1/1  "<q_bar>"
  Gain1/1 -> Add/5
  Bus Selector/5 -> Gain/1  "<alphadot>"
  Gain/1 -> Add/4
  Bus Selector/4 -> CLde/1  "<de>"
  CLde/1 -> Add/3
  Add/1 -> Product/1
  Product/1 -> CL/1
  Groud Effect Look Up/1 -> Product/2
  Gain2/1 -> Saturation/1
  Saturation/1 -> Groud Effect Look Up/1
  Bus Selector/7 -> Gain2/1  "<realtive height>"
  Sum/1 -> Add/1
  CLalpha0/1 -> Sum/2
  Bus Selector/1 -> Gain3/1  "<alpha>"
  Gain3/1 -> Sum/1
  Bus Selector/2 -> Terminator/1  "<beta>"
  Bus Selector/3 -> Product1/2, Product1/1, Gain5/1  "<flap>"
  Sum1/1 -> Add/2
  Gain4/1 -> Sum1/1
  Gain5/1 -> Sum1/2
  Product1/1 -> Gain4/1

== system kinematicstest/Aerodynamic Force and Moments/Aerodynamic Force /Side Coefficient ==
  aero_input : Inport
  Bus Selector : BusSelector  OutputSignals=r_bar,p_bar,dr,da,beta
  CYbeta : Gain  Gain=C172.Aerodynamics.Side.CYb
  CYbeta1 : Gain  Gain=C172.Aerodynamics.Side.CYda
  CYbeta2 : Gain  Gain=C172.Aerodynamics.Side.CYdr
  CYbeta3 : Gain  Gain=C172.Aerodynamics.Side.CYp
  CYbeta4 : Gain  Gain=C172.Aerodynamics.Side.CYr
  Sum : Sum  Inputs=+++++
  CY : Outport
  wires:
  Sum/1 -> CY/1
  aero_input/1 -> Bus Selector/1
  CYbeta/1 -> Sum/5
  CYbeta1/1 -> Sum/4
  CYbeta2/1 -> Sum/3
  CYbeta3/1 -> Sum/2
  CYbeta4/1 -> Sum/1
  Bus Selector/1 -> CYbeta4/1  "<r_bar>"
  Bus Selector/2 -> CYbeta3/1  "<p_bar>"
  Bus Selector/3 -> CYbeta2/1  "<dr>"
  Bus Selector/4 -> CYbeta1/1  "<da>"
  Bus Selector/5 -> CYbeta/1  "<beta>"

== system kinematicstest/Aerodynamic Force and Moments/Aerodynamic Moments/Cl ==
  note: C172.Aerodynamics.Roll.Clb = -0.0891;%rad
      | C172.Aerodynamics.Roll.Clp = -0.47;% p-aero-rad_sec bi2vel
      | C172.Aerodynamics.Roll.Clr.Rowalpha = [0 0.094];  %rad
      | C172.Aerodynamics.Roll.Clr.Table = [0.08 0.19];   %rad
      | C172.Aerodynamics.Roll.Clda = 0.23;% rad
      | C172.Aerodynamics.Roll.Cldr = 0.0147;% rad
  aero_input : Inport
  1-D Lookup Table : Lookup_n-D  NumberOfTableDimensions=1  BreakpointsForDimension1=C172.Aerodynamics.Roll.Clr.Rowalpha  Table=C172.Aerodynamics.Roll.Clr.Table  InternalRulePriority=Speed  RndMeth=Simplest  InputSameDT=on
  Add : Sum  Inputs=+++++
  Bus Selector : BusSelector  OutputSignals=beta,p_bar,r_bar,alpha,da,dr
  Gain : Gain  Gain=C172.Aerodynamics.Roll.Clb
  Gain1 : Gain  Gain=C172.Aerodynamics.Roll.Clp
  Gain2 : Gain  Gain=C172.Aerodynamics.Roll.Clda
  Gain3 : Gain  Gain=C172.Aerodynamics.Roll.Cldr
  Product6 : Product  RndMeth=Zero
  Saturation : Saturate  UpperLimit=0.05  LowerLimit=-0.05
  Cl : Outport
  wires:
  aero_input/1 -> Bus Selector/1
  Add/1 -> Cl/1
  Bus Selector/3 -> Product6/1  "<r_bar>"
  1-D Lookup Table/1 -> Product6/2
  Gain/1 -> Saturation/1
  Gain1/1 -> Add/2
  Product6/1 -> Add/3
  Saturation/1 -> Add/1
  Bus Selector/1 -> Gain/1  "<beta>"
  Bus Selector/2 -> Gain1/1  "<p_bar>"
  Bus Selector/4 -> 1-D Lookup Table/1  "<alpha>"
  Bus Selector/5 -> Gain2/1  "<da>"
  Gain2/1 -> Add/4
  Bus Selector/6 -> Gain3/1  "<dr>"
  Gain3/1 -> Add/5

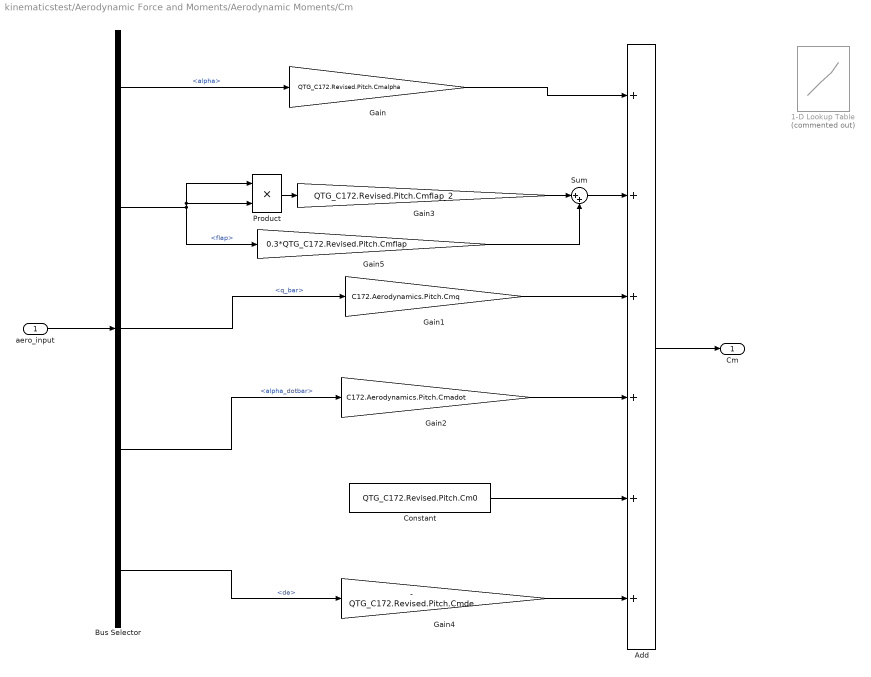
== system kinematicstest/Aerodynamic Force and Moments/Aerodynamic Moments/Cm ==
  aero_input : Inport
  1-D Lookup Table : Lookup_n-D  Commented=on  NumberOfTableDimensions=1  BreakpointsForDimension1=C172.Aerodynamics.Pitch.CmDf.RowFlap  Table=C172.Aerodynamics.Pitch.CmDf.Table  InternalRulePriority=Speed  RndMeth=Simplest  InputSameDT=on
  Add : Sum  Inputs=++++++
  Bus Selector : BusSelector  OutputSignals=alpha,flap,q_bar,alpha_dotbar,de
  Constant : Constant  Value=QTG_C172.Revised.Pitch.Cm0
  Gain : Gain  Gain=QTG_C172.Revised.Pitch.Cmalpha
  Gain1 : Gain  Gain=C172.Aerodynamics.Pitch.Cmq
  Gain2 : Gain  Gain=C172.Aerodynamics.Pitch.Cmadot
  Gain3 : Gain  Gain=QTG_C172.Revised.Pitch.Cmflap_2
  Gain4 : Gain  Gain=- QTG_C172.Revised.Pitch.Cmde
  Gain5 : Gain  Gain=0.3*QTG_C172.Revised.Pitch.Cmflap
  Product : Product
  Sum : Sum  Inputs=|++
  Cm : Outport
  wires:
  Add/1 -> Cm/1
  aero_input/1 -> Bus Selector/1
  Bus Selector/1 -> Gain/1  "<alpha>"
  Gain1/1 -> Add/3
  Gain/1 -> Add/1
  Gain2/1 -> Add/4
  Constant/1 -> Add/5
  Gain4/1 -> Add/6
  Bus Selector/3 -> Gain1/1  "<q_bar>"
  Bus Selector/4 -> Gain2/1  "<alpha_dotbar>"
  Bus Selector/5 -> Gain4/1  "<de>"
  Sum/1 -> Add/2
  Product/1 -> Gain3/1
  Gain3/1 -> Sum/1
  Gain5/1 -> Sum/2
  Bus Selector/2 -> Product/2, Product/1, Gain5/1  "<flap>"

== system kinematicstest/Aerodynamic Force and Moments/Aerodynamic Moments/Cn ==
  note: C172.Aerodynamics.Yaw.Cnb = 0.0650;% rad
      | C172.Aerodynamics.Yaw.Cnp = -0.03;% p-aero-rad_sec bi2vel
      | C172.Aerodynamics.Yaw.Cnr = -0.099;%  r-aero-rad_sec bi2vel
      | C172.Aerodynamics.Yaw.Cnda = 0.0053;% rad
      | C172.Aerodynamics.Yaw.Cndr = -0.043;% rad
  aero_input : Inport
  Add : Sum  Inputs=+++++
  Bus Selector : BusSelector  OutputSignals=beta,p_bar,r_bar,da,dr
  Cnp : Gain  Gain=C172.Aerodynamics.Yaw.Cnp
  Cnp1 : Gain  Gain=C172.Aerodynamics.Yaw.Cnr
  Cnp2 : Gain  Gain=C172.Aerodynamics.Yaw.Cnda
  Cnp3 : Gain  Gain=C172.Aerodynamics.Yaw.Cndr
  Gain : Gain  Gain=C172.Aerodynamics.Yaw.Cnb
  Cn : Outport
  wires:
  aero_input/1 -> Bus Selector/1
  Add/1 -> Cn/1
  Bus Selector/3 -> Cnp1/1  "<r_bar>"
  Bus Selector/4 -> Cnp2/1  "<da>"
  Bus Selector/1 -> Gain/1  "<beta>"
  Gain/1 -> Add/1
  Cnp/1 -> Add/2
  Bus Selector/2 -> Cnp/1  "<p_bar>"
  Cnp1/1 -> Add/3
  Cnp2/1 -> Add/4
  Cnp3/1 -> Add/5
  Bus Selector/5 -> Cnp3/1  "<dr>"

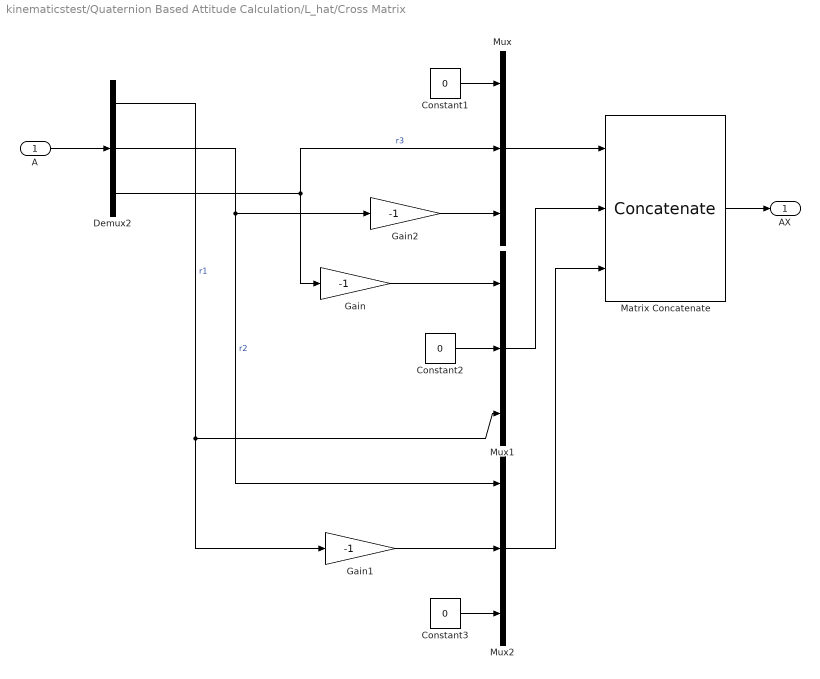
== system kinematicstest/Quaternion Based Attitude Calculation/L_hat/Cross Matrix ==
  A : Inport
  Constant1 : Constant  Value=0
  Constant2 : Constant  Value=0
  Constant3 : Constant  Value=0
  Demux2 : Demux  Outputs=3
  Gain : Gain  Gain=-1
  Gain1 : Gain  Gain=-1
  Gain2 : Gain  Gain=-1
  Matrix Concatenate : Concatenate  NumInputs=3  Mode=Multidimensional array  ConcatenateDimension=2
  Mux : Mux  Inputs=3
  Mux1 : Mux  Inputs=3
  Mux2 : Mux  Inputs=3
  AX : Outport
  wires:
  A/1 -> Demux2/1
  Demux2/1 -> Mux1/3, Gain1/1  "r1"
  Demux2/2 -> Mux2/1, Gain2/1  "r2"
  Matrix Concatenate/1 -> AX/1
  Demux2/3 -> Gain/1, Mux/2  "r3"
  Mux/1 -> Matrix Concatenate/1
  Mux1/1 -> Matrix Concatenate/2
  Constant2/1 -> Mux1/2
  Gain/1 -> Mux1/1
  Mux2/1 -> Matrix Concatenate/3
  Gain1/1 -> Mux2/2
  Constant3/1 -> Mux2/3
  Constant1/1 -> Mux/1
  Gain2/1 -> Mux/3
